simulink model "mod_prj"  (R2019b)
settings: Solver=VariableStepAuto  StartTime=0.0  StopTime=10.0  RelTol=1e-3
values from neighbouring files (symbols this model uses):
  m = 6    [meanValueAnalysis.m]
undefined symbols (not defined in the file or in its folder): n
libraries: dspsrcs4 x2
settings Model: Creator=aadi0  LastModifiedBy=aadi0

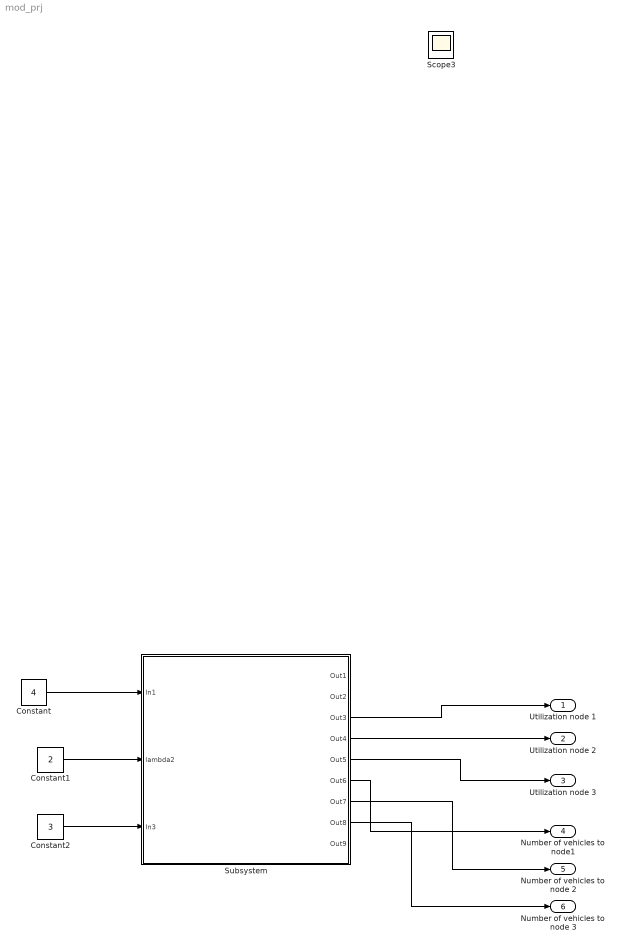
== system mod_prj ==
  Constant : Constant  Value=4
  Constant1 : Constant  Value=2
  Constant2 : Constant  Value=3
  Subsystem : Subsystem
  Utilization node 1 : Outport
  Utilization node 2 : Outport  Port=2
  Utilization node 3 : Outport  Port=3
  Number of vehicles to node1 : Outport  Port=4
  Number of vehicles to node 2 : Outport  Port=5
  Number of vehicles to node 3 : Outport  Port=6
  Scope3 : Scope
  wires:
  Constant/1 -> Subsystem/1(In1)
  Constant1/1 -> Subsystem/2(lambda2)
  Constant2/1 -> Subsystem/3(In3)
  Subsystem/3(Out3) -> Utilization node 1/1
  Subsystem/4(Out4) -> Utilization node 2/1
  Subsystem/5(Out5) -> Utilization node 3/1
  Subsystem/6(Out6) -> Number of vehicles to node1/1
  Subsystem/7(Out7) -> Number of vehicles to node 2/1
  Subsystem/8(Out8) -> Number of vehicles to node 3/1

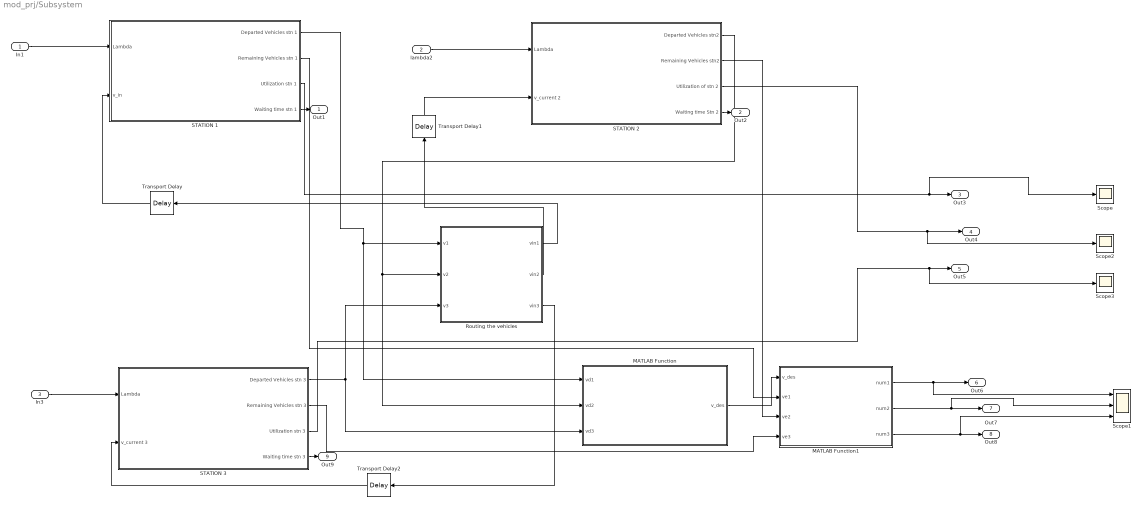
== system mod_prj/Subsystem ==
  In1 : Inport
  lambda2 : Inport  Port=2
  In3 : Inport  Port=3
  MATLAB Function : MATLAB Function  TreatAsAtomicUnit=on
  MATLAB Function1 : MATLAB Function  TreatAsAtomicUnit=on
  "Routing the vehicles " : MATLAB Function  TreatAsAtomicUnit=on
  STATION 1 : Subsystem
  STATION 2 : Subsystem
  STATION 3 : Subsystem
  Scope : Scope
  Scope1 : Scope  NumInputPorts=3
  Scope2 : Scope
  Scope3 : Scope
  Transport Delay : TransportDelay  DelayTime=2
  Transport Delay1 : TransportDelay  DelayTime=3
  Transport Delay2 : TransportDelay
  Out1 : Outport
  Out2 : Outport  Port=2
  Out3 : Outport  Port=3
  Out4 : Outport  Port=4
  Out5 : Outport  Port=5
  Out6 : Outport  Port=6
  Out7 : Outport  Port=7
  Out8 : Outport  Port=8
  Out9 : Outport  Port=9
  wires:
  Transport Delay/1 -> STATION 1/2("v_in ")
  STATION 3/1(Departed Vehicles stn 3) -> "Routing the vehicles "/3(v3), MATLAB Function/3(vd3)
  STATION 2/1(Departed Vehicles stn2) -> MATLAB Function/2(vd2), "Routing the vehicles "/2(v2)
  STATION 1/1(Departed Vehicles stn 1) -> MATLAB Function/1(vd1), "Routing the vehicles "/1(v1)
  "Routing the vehicles "/2(vin2) -> Transport Delay1/1
  STATION 1/4("Waiting time stn 1 ") -> Out1/1
  Transport Delay1/1 -> STATION 2/2("v_current 2 ")
  MATLAB Function1/2(num2) -> Scope1/2, Out7/1
  "Routing the vehicles "/1(vin1) -> Transport Delay/1
  STATION 2/2("Remaining Vehicles stn2 ") -> MATLAB Function1/3(ve2)
  STATION 1/2(Remaining Vehicles stn 1) -> MATLAB Function1/2(ve1)
  "Routing the vehicles "/3(vin3) -> Transport Delay2/1
  MATLAB Function/1(v_des) -> MATLAB Function1/1(v_des)
  Transport Delay2/1 -> STATION 3/2(v_current 3)
  In1/1 -> STATION 1/1(Lambda)
  lambda2/1 -> STATION 2/1(Lambda)
  STATION 3/2(Remaining Vehicles stn 3) -> MATLAB Function1/4(ve3)
  In3/1 -> STATION 3/1(Lambda)
  STATION 2/3("Utilization of stn 2 ") -> Scope2/1, Out4/1
  STATION 3/3(Utilization stn 3) -> Scope3/1, Out5/1
  STATION 2/4(Waiting time Stn 2) -> Out2/1
  MATLAB Function1/1(num1) -> Scope1/1, Out6/1
  MATLAB Function1/3(num3) -> Scope1/3, Out8/1
  STATION 1/3("Utilization stn 1 ") -> Scope/1, Out3/1
  STATION 3/4(Waiting time stn 3) -> Out9/1

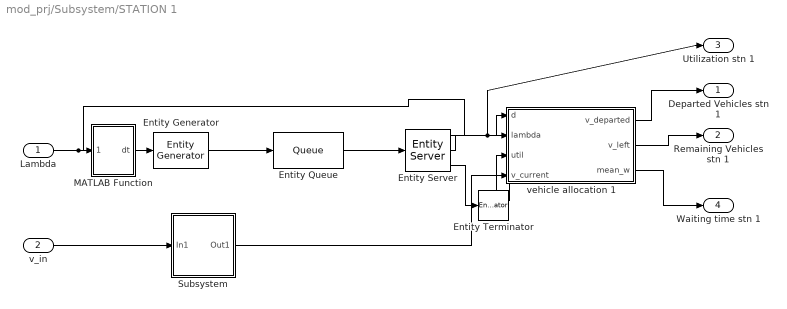
== system mod_prj/Subsystem/STATION 1 ==
  Lambda : Inport
  "v_in " : Inport  Port=2
  Entity Generator : EntityGenerator  OutputPortMessageModes=m  TimeSource=Signal port  Period=2  IntergenerationTimeAction=dt = poissrnd(lambda,1);  AttributeName=Customer_stn1  EntityType=Structured  EntityTypeName=Entity
      settings: InputPortMap=u1
  Entity Queue : Queue  InputPortMessageModes=m  OutputPortMessageModes=m  Capacity=10
  Entity Server : EntityServer  InputPortMessageModes=m  OutputPortMessageModes=n,n,m  Capacity=1  ServiceTimeValue=0.2  NumberEntitiesDeparted=on  Utilization=on
      settings: OutputPortMap=o0,o5,o9
  Entity Terminator : EntityTerminator  InputPortMessageModes=m
  MATLAB Function : MATLAB Function  TreatAsAtomicUnit=on
  Subsystem : Subsystem
  "vehicle allocation 1 " : MATLAB Function  TreatAsAtomicUnit=on
  Departed Vehicles stn 1 : Outport
  Remaining Vehicles stn 1 : Outport  Port=2
  "Utilization stn 1 " : Outport  Port=3
  "Waiting time stn 1 " : Outport  Port=4
  wires:
  Entity Generator/1 -> Entity Queue/1
  Entity Server/3 -> Entity Terminator/1
  Entity Queue/1 -> Entity Server/1
  Entity Server/1 -> "vehicle allocation 1 "/1(d)
  "vehicle allocation 1 "/2(v_left) -> Remaining Vehicles stn 1/1
  Entity Server/2 -> "vehicle allocation 1 "/3(util), "Utilization stn 1 "/1
  Lambda/1 -> "vehicle allocation 1 "/2(lambda), MATLAB Function/1(lambda)
  "vehicle allocation 1 "/1(v_departed) -> Departed Vehicles stn 1/1
  "vehicle allocation 1 "/3(mean_w) -> "Waiting time stn 1 "/1
  MATLAB Function/1(dt) -> Entity Generator/1
  "v_in "/1 -> Subsystem/1(In1)
  Subsystem/1(Out1) -> "vehicle allocation 1 "/4(v_current)

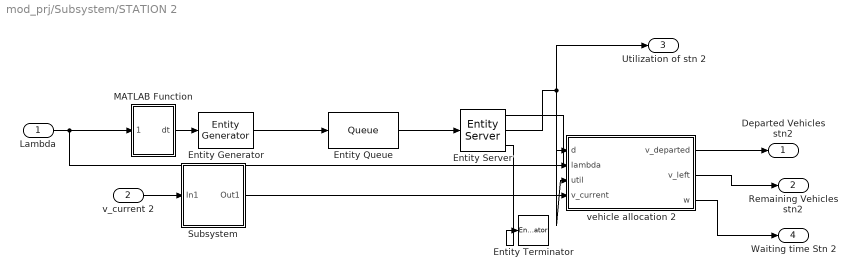
== system mod_prj/Subsystem/STATION 2 ==
  Lambda : Inport
  "v_current 2 " : Inport  Port=2
  Entity Generator : EntityGenerator  OutputPortMessageModes=m  TimeSource=Signal port  Period=2  AttributeName=Customer_stn1  EntityType=Structured  EntityTypeName=Entity
      settings: InputPortMap=u1
  Entity Queue : Queue  InputPortMessageModes=m  OutputPortMessageModes=m  Capacity=6
  Entity Server : EntityServer  InputPortMessageModes=m  OutputPortMessageModes=n,n,m  Capacity=1  ServiceTimeValue=0.5  NumberEntitiesDeparted=on  Utilization=on
      settings: OutputPortMap=o0,o5,o9
  Entity Terminator : EntityTerminator  InputPortMessageModes=m
  MATLAB Function : MATLAB Function  TreatAsAtomicUnit=on
  Subsystem : Subsystem
  "vehicle allocation 2 " : MATLAB Function  TreatAsAtomicUnit=on
  Departed Vehicles stn2 : Outport
  "Remaining Vehicles stn2 " : Outport  Port=2
  "Utilization of stn 2 " : Outport  Port=3
  Waiting time Stn 2 : Outport  Port=4
  wires:
  "vehicle allocation 2 "/1(v_departed) -> Departed Vehicles stn2/1
  Entity Server/2 -> "vehicle allocation 2 "/3(util), "Utilization of stn 2 "/1
  "vehicle allocation 2 "/2(v_left) -> "Remaining Vehicles stn2 "/1
  Entity Server/1 -> "vehicle allocation 2 "/1(d)
  Entity Queue/1 -> Entity Server/1
  Entity Server/3 -> Entity Terminator/1
  Entity Generator/1 -> Entity Queue/1
  Lambda/1 -> MATLAB Function/1(lambda), "vehicle allocation 2 "/2(lambda)
  "vehicle allocation 2 "/3(w) -> Waiting time Stn 2/1
  MATLAB Function/1(dt) -> Entity Generator/1
  "v_current 2 "/1 -> Subsystem/1(In1)
  Subsystem/1(Out1) -> "vehicle allocation 2 "/4(v_current)

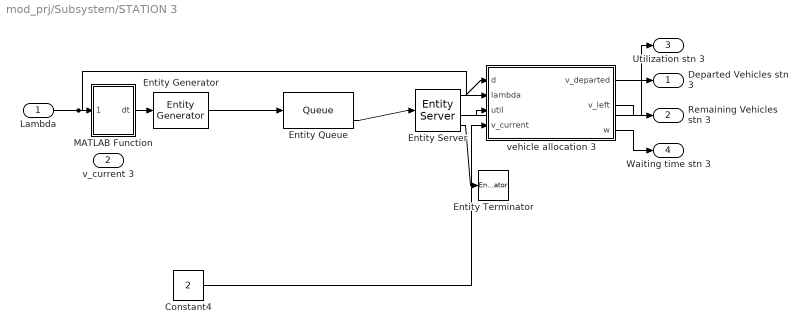
== system mod_prj/Subsystem/STATION 3 ==
  Lambda : Inport
  v_current 3 : Inport  Port=2
  Constant4 : Constant  Value=2
  Entity Generator : EntityGenerator  OutputPortMessageModes=m  TimeSource=Signal port  Period=2  AttributeName=Customer_stn1  EntityType=Structured  EntityTypeName=Entity
      settings: InputPortMap=u1
  Entity Queue : Queue  InputPortMessageModes=m  OutputPortMessageModes=n,m  Capacity=8  AverageWait=on
      settings: OutputPortMap=o2,o5
  Entity Server : EntityServer  InputPortMessageModes=m  OutputPortMessageModes=n,n,n,m  Capacity=1  ServiceTimeValue=1  NumberEntitiesDeparted=on  NumberEntitiesInBlock=on  Utilization=on
      settings: OutputPortMap=o0,o1,o5,o9
  Entity Terminator : EntityTerminator  InputPortMessageModes=m
  MATLAB Function : MATLAB Function  TreatAsAtomicUnit=on
  vehicle allocation 3 : MATLAB Function  TreatAsAtomicUnit=on
  Departed Vehicles stn 3 : Outport
  Remaining Vehicles stn 3 : Outport  Port=2
  Utilization stn 3 : Outport  Port=3
  Waiting time stn 3 : Outport  Port=4
  wires:
  Entity Generator/1 -> Entity Queue/1
  Entity Server/4 -> Entity Terminator/1
  Entity Queue/2 -> Entity Server/1
  Entity Server/1 -> vehicle allocation 3/1(d)
  vehicle allocation 3/2(v_left) -> Remaining Vehicles stn 3/1
  Entity Server/3 -> vehicle allocation 3/3(util), Utilization stn 3/1
  Lambda/1 -> vehicle allocation 3/2(lambda), MATLAB Function/1(lambda)
  vehicle allocation 3/1(v_departed) -> Departed Vehicles stn 3/1
  vehicle allocation 3/3(w) -> Waiting time stn 3/1
  MATLAB Function/1(dt) -> Entity Generator/1
  Constant4/1 -> vehicle allocation 3/4(v_current)

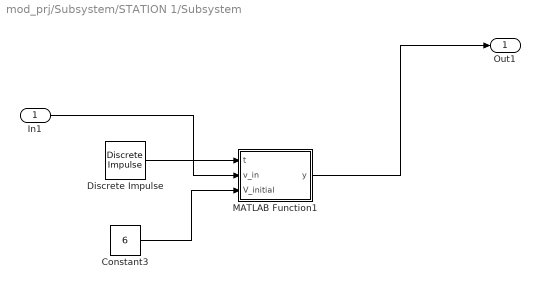
== system mod_prj/Subsystem/STATION 1/Subsystem ==
  In1 : Inport
  Constant3 : Constant  Value=6
  Discrete Impulse : dspsrcs4/Discrete  Impulse  Delay=0  SampleTime=1  FrameSample=1  OutputFrames=off  dataType=double  isSigned=on  wordLen=16  udDataType=sfix(16)  fracBitsMode=Best precision  numFracBits=15  OutDataTypeStr=double  LastOutDataTypeStr=double
  MATLAB Function1 : MATLAB Function  TreatAsAtomicUnit=on
  Out1 : Outport
  wires:
  Discrete Impulse/1 -> MATLAB Function1/1(t)
  In1/1 -> MATLAB Function1/2(v_in)
  Constant3/1 -> MATLAB Function1/3(V_initial)
  MATLAB Function1/1(y) -> Out1/1

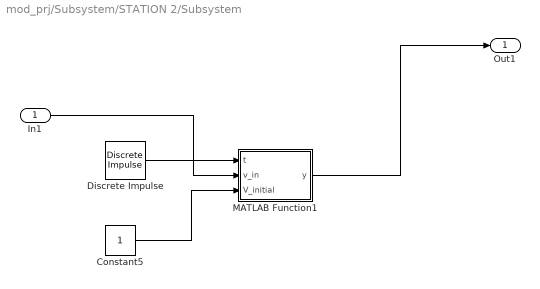
== system mod_prj/Subsystem/STATION 2/Subsystem ==
  In1 : Inport
  Constant5 : Constant
  Discrete Impulse : dspsrcs4/Discrete  Impulse  Delay=0  SampleTime=1  FrameSample=1  OutputFrames=off  dataType=double  isSigned=on  wordLen=16  udDataType=sfix(16)  fracBitsMode=Best precision  numFracBits=15  OutDataTypeStr=double  LastOutDataTypeStr=double
  MATLAB Function1 : MATLAB Function  TreatAsAtomicUnit=on
  Out1 : Outport
  wires:
  Discrete Impulse/1 -> MATLAB Function1/1(t)
  In1/1 -> MATLAB Function1/2(v_in)
  Constant5/1 -> MATLAB Function1/3(V_initial)
  MATLAB Function1/1(y) -> Out1/1

== matlab function mod_prj/Subsystem/STATION 2/vehicle allocation 2  ==
  data: d input; v_departed output; v_left output; lambda input; util input; v_current input; w output
function [v_departed,v_left,w] = vServer(d,lambda,util,v_current)
w = lambda/util;
if v_current>d
    v_departed  = d;
    v_left = v_current-v_departed;
    
else
    v_departed = v_current;
    v_left = 0;
    
end

== matlab function mod_prj/Subsystem/STATION 1/vehicle allocation 1  ==
  data: d input; lambda input; v_departed output; v_left output; util input; v_current input; mean_w output
function [v_departed,v_left,mean_w] = vServer(d,lambda,util,v_current)
mean_w =  (lambda/util*v_current);
if v_current>d
    v_departed  = d;
    v_left = v_current-v_departed;
    
else
    v_departed = v_current;
    v_left = 0;
    
end

== matlab function mod_prj/Subsystem/STATION 3/vehicle allocation 3 ==
  data: d input; v_departed output; v_left output; lambda input; util input; v_current input; w output
function [v_departed,v_left,w] = vServer(d,lambda,util,v_current)
w = lambda/util;
if v_current>d
    v_departed  = d;
    v_left = v_current-v_departed;
    
else
    v_departed = v_current;
    v_left = 0;
    
end

== matlab function mod_prj/Subsystem/Routing the vehicles  ==
  data: v1 input; vin1 output; v2 input; v3 input; vin2 output; vin3 output
function [vin1, vin2, vin3] = vRouting(v1,v2,v3)
P = [0 0.4 0.6;
    0.5 0 0.5;
    0.3 0.7 0];
v_route = zeros(3);
vout = [v1,v2,v3];
for i = 1:3
    for j = 1:3
        v_route(i,j) = P(i,j)*vout(i);
    end
end
vin1 = round(v_route(2,1))+round(v_route(3,1));
vin2 = round(v_route(1,2))+round(v_route(3,2));
vin3 = round(v_route(1,3))+round(v_route(2,3));

== matlab function mod_prj/Subsystem/STATION 1/MATLAB Function ==
  data: lambda input; dt output
function dt = fcn(lambda)

dt = poissrnd(lambda);

== matlab function mod_prj/Subsystem/STATION 3/MATLAB Function ==
  data: lambda input; dt output
function dt = fcn(lambda)

dt = poissrnd(lambda);

== matlab function mod_prj/Subsystem/STATION 2/MATLAB Function ==
  data: lambda input; dt output
function dt = fcn(lambda)

dt = poissrnd(lambda);

== matlab function mod_prj/Subsystem/MATLAB Function ==
  data: vd1 input; vd2 input; vd3 input; v_des output
function v_des = desiredVehicles(vd1,vd2,vd3)
v_dep = [vd1,vd2,vd3];
m = 15;
sum = 0;
for i = 1:3
    sum = sum + v_dep(i);
end
vx_total = m - sum;
v_des = vx_total/3;

== matlab function mod_prj/Subsystem/STATION 1/Subsystem/MATLAB Function1 ==
  data: t input; y output; v_in input; V_initial input
function y = input(t,v_in,V_initial)
if t == 1
    y = V_initial;
else
    y = v_in;
end

== matlab function mod_prj/Subsystem/STATION 2/Subsystem/MATLAB Function1 ==
  data: t input; y output; v_in input; V_initial input
function y = input(t,v_in,V_initial)
if t == 1
    y = V_initial;
else
    y = v_in;
end

== matlab function mod_prj/Subsystem/MATLAB Function1 ==
  data: v_des input; num1 output; ve1 input; ve2 input; ve3 input; num2 output; num3 output
function [num1, num2, num3] = rebalancingVehicles(v_des, ve1,ve2,ve3)
%linearly optimizing the number of vehicles to a station
n1 = max(v_des-ve1);
n2 = max(v_des-ve2);
n3 = max(v_des-ve3);
if n1<0
    num1 = 0;
else 
    num1 = round(n1);
end
if n2<0
    num2 = 0;
else 
    num2 = round(n2);
end
if n3<0
    num3 = 0;
else 
    num3 = round(n3);
end
